simulink model "Mai9lab"  (R2020a)
settings: Solver=VariableStepAuto  StartTime=0.0  StopTime=52  RelTol=1e-3
settings Model: SimulationMode=accelerator  PacingRate=18  Creator=thang_mai  LastModifiedBy=thang_mai

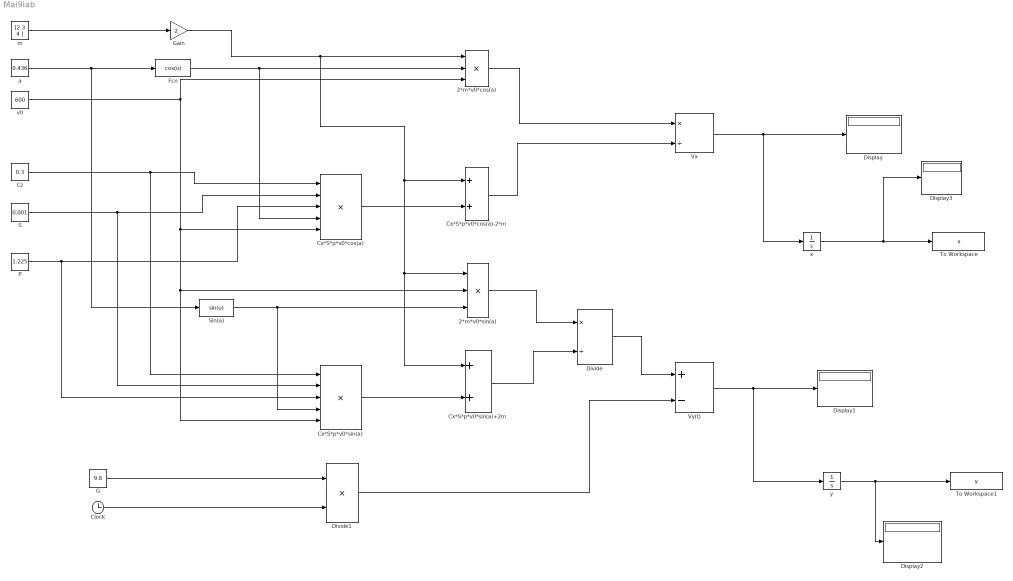
== system Mai9lab ==
  2*m*v0*cos(a) : Product  Inputs=***
  2*m*v0*sin(a) : Product  Inputs=***
  Clock : Clock
      settings: Decimation=52
  Cx*S*p*v0*cos(a) : Product  Inputs=*****
  Cx*S*p*v0*cos(a)-2*m : Sum
  Cx*S*p*v0*sin(a) : Product  Inputs=*****
  Cx*S*p*v0*sin(a)+2m : Sum
  Cz : Constant  Value=0.3
  Display{,1..3} (4 alike) : Display
  Divide : Product  Inputs=*/
  Divide1 : Product  Inputs=**
  Fcn : Fcn  Expr=cos(u)
  G : Constant  Value=9.8
  Gain : Gain  Gain=2
  P : Constant  Value=1.225
  S : Constant  Value=0.001
  Sin(a) : Fcn  Expr=sin(u)
  To Workspace : ToWorkspace  VariableName=x  SampleTime=-1
      settings: Save2DSignal=2-D array (concatenate along first dimension)
  To Workspace1 : ToWorkspace  VariableName=y  SampleTime=-1
      settings: Save2DSignal=2-D array (concatenate along first dimension)
  Vx : Product  Inputs=*/
  Vy(t) : Sum  Inputs=+-
  a : Constant  Value=0.436
  m : Constant  Value=[2 3 4 ]  VectorParams1D=off
  v0 : Constant  Value=600
  x : Integrator
  y : Integrator
  wires:
  m/1 -> Gain/1
  a/1 -> Sin(a)/1, Fcn/1
  Fcn/1 -> Cx*S*p*v0*cos(a)/4, 2*m*v0*cos(a)/2
  Cx*S*p*v0*cos(a)/1 -> Cx*S*p*v0*cos(a)-2*m/2
  2*m*v0*cos(a)/1 -> Vx/1
  Cx*S*p*v0*cos(a)-2*m/1 -> Vx/2
  Vx/1 -> x/1, Display/1
  S/1 -> Cx*S*p*v0*sin(a)/2, Cx*S*p*v0*cos(a)/2
  Sin(a)/1 -> Cx*S*p*v0*sin(a)/4, 2*m*v0*sin(a)/3
  P/1 -> Cx*S*p*v0*cos(a)/3, Cx*S*p*v0*sin(a)/3
  Cz/1 -> Cx*S*p*v0*sin(a)/1, Cx*S*p*v0*cos(a)/1
  v0/1 -> 2*m*v0*cos(a)/3, Cx*S*p*v0*sin(a)/5, 2*m*v0*sin(a)/2, Cx*S*p*v0*cos(a)/5
  Cx*S*p*v0*sin(a)/1 -> Cx*S*p*v0*sin(a)+2m/2
  Gain/1 -> Cx*S*p*v0*sin(a)+2m/1, 2*m*v0*sin(a)/1, Cx*S*p*v0*cos(a)-2*m/1, 2*m*v0*cos(a)/1
  2*m*v0*sin(a)/1 -> Divide/1
  Cx*S*p*v0*sin(a)+2m/1 -> Divide/2
  Divide/1 -> Vy(t)/1
  G/1 -> Divide1/1
  Vy(t)/1 -> y/1, Display1/1
  x/1 -> To Workspace/1, Display3/1
  y/1 -> Display2/1, To Workspace1/1
  Clock/1 -> Divide1/2
  Divide1/1 -> Vy(t)/2
